simulink model "KeyboardControl_2017a"  (R2017a)
settings: Solver=FixedStepAuto  StartTime=0.0  StopTime=inf  FixedStep=Ts  RelTol=1e-3
libraries: instrumentlib x1
settings Model: Creator=jakubkryczka  LastModifiedBy=thh206

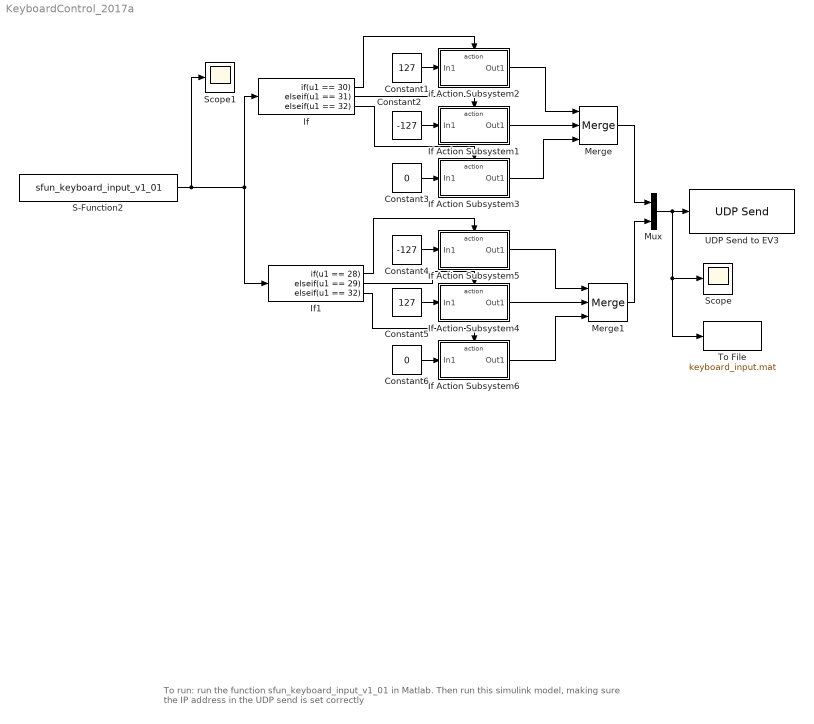
== system KeyboardControl_2017a ==
  note: To run: run the function sfun_keyboard_input_v1_01 in Matlab. Then run this simulink model, making sure the IP address in the UDP send is set correctly
  Constant1 : Constant  Value=127
  Constant2 : Constant  Value=-127
  Constant3 : Constant  Value=0
  Constant4 : Constant  Value=-127
  Constant5 : Constant  Value=127
  Constant6 : Constant  Value=0
  If : If  IfExpression=u1 == 30  ElseIfExpressions=u1 == 31,u1 == 32  ShowElse=off
  If Action Subsystem1 : Subsystem  TreatAsAtomicUnit=on
  If Action Subsystem2 : Subsystem  TreatAsAtomicUnit=on
  If Action Subsystem3 : Subsystem  TreatAsAtomicUnit=on
  If Action Subsystem4 : Subsystem  TreatAsAtomicUnit=on
  If Action Subsystem5 : Subsystem  TreatAsAtomicUnit=on
  If Action Subsystem6 : Subsystem  TreatAsAtomicUnit=on
  If1 : If  IfExpression=u1 == 28  ElseIfExpressions=u1 == 29,u1 == 32  ShowElse=off
  Merge : Merge  Inputs=3  InitialOutput=0
  Merge1 : Merge  Inputs=3  InitialOutput=0
  Mux : Mux  Inputs=2
  S-Function2 : S-Function  FunctionName=sfun_keyboard_input_v1_01  Parameters=Ts  SFunctionDeploymentMode=off  EnableBusSupport=off
  Scope : Scope
  Scope1 : Scope
  To File : ToFile  Filename=keyboard_input.mat  MatrixName=keyboard_input
  UDP Send to EV3 : instrumentlib/UDP Send  Host=192.168.1.3  Port=25000  LocalPort=-1  EnablePortSharing=off  ByteOrder=LittleEndian  OutputDatagramPacketSize=512  EnableBlockingMode=off  LocalAddress=0.0.0.0
      settings: SourceProductName=Instrument Control Toolbox
  wires:
  Merge/1 -> Mux/1
  Constant2/1 -> If Action Subsystem1/1(In1)
  If Action Subsystem2/1(Out1) -> Merge/1
  Constant1/1 -> If Action Subsystem2/1(In1)
  If/3 -> If Action Subsystem3/Action
  If/2 -> If Action Subsystem1/Action
  If/1 -> If Action Subsystem2/Action
  Constant3/1 -> If Action Subsystem3/1(In1)
  Constant6/1 -> If Action Subsystem6/1(In1)
  If1/2 -> If Action Subsystem4/Action
  Constant4/1 -> If Action Subsystem5/1(In1)
  If1/1 -> If Action Subsystem5/Action
  If Action Subsystem5/1(Out1) -> Merge1/1
  S-Function2/1 -> Scope1/1, If1/1, If/1
  Constant5/1 -> If Action Subsystem4/1(In1)
  If1/3 -> If Action Subsystem6/Action
  Merge1/1 -> Mux/2
  Mux/1 -> To File/1, Scope/1, UDP Send to EV3/1
  If Action Subsystem1/1(Out1) -> Merge/2
  If Action Subsystem3/1(Out1) -> Merge/3
  If Action Subsystem4/1(Out1) -> Merge1/2
  If Action Subsystem6/1(Out1) -> Merge1/3

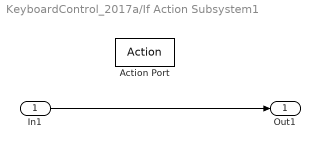
== system KeyboardControl_2017a/If Action Subsystem1 ==
  In1 : Inport
  Action Port : ActionPort
  Out1 : Outport
  wires:
  In1/1 -> Out1/1

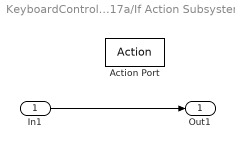
== system KeyboardControl_2017a/If Action Subsystem2 ==
  In1 : Inport
  Action Port : ActionPort
  Out1 : Outport
  wires:
  In1/1 -> Out1/1

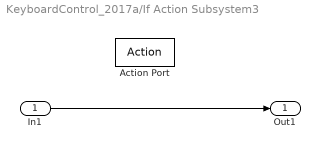
== system KeyboardControl_2017a/If Action Subsystem3 ==
  In1 : Inport
  Action Port : ActionPort
  Out1 : Outport
  wires:
  In1/1 -> Out1/1

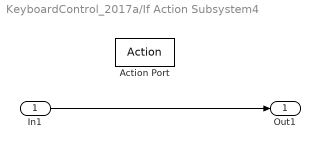
== system KeyboardControl_2017a/If Action Subsystem4 ==
  In1 : Inport
  Action Port : ActionPort
  Out1 : Outport
  wires:
  In1/1 -> Out1/1

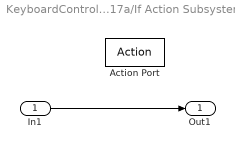
== system KeyboardControl_2017a/If Action Subsystem5 ==
  In1 : Inport
  Action Port : ActionPort
  Out1 : Outport
  wires:
  In1/1 -> Out1/1

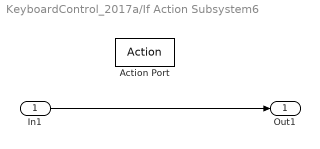
== system KeyboardControl_2017a/If Action Subsystem6 ==
  In1 : Inport
  Action Port : ActionPort
  Out1 : Outport
  wires:
  In1/1 -> Out1/1
